simulink model "MLRC_Project_debug"  (R2022a)
settings: Solver=ode45  StartTime=0.0  StopTime=100  RelTol=1e-3  EnableMultiTasking=on
settings Model: Creator=Administrator  LastModifiedBy=rakes
settings DataIOCC: LimitDataPoints=on  SaveFormat=Array  ReturnWorkspaceOutputs=off
settings OptimizationCC: LifeSpan=inf
settings DebuggingCC: SolverPrmCheckMsg=warning  UnconnectedInputMsg=warning  UnconnectedOutputMsg=warning  UnconnectedLineMsg=warning  AllowSymbolicDim=off  SFUnexpectedBacktrackingDiag=warning  SFNoUnconditionalDefaultTransitionDiag=warning  SFExecutionAtInitializationDiag=none  SFMachineParentedDataDiag=warning  ArithmeticOperatorsInVariantConditions=warning
settings HardwareCC: ProdBitPerPointer=32  ProdBitPerSizeT=32  ProdBitPerPtrDiffT=32  ProdLargestAtomicFloat=None  ProdIntDivRoundTo=Undefined  ProdEndianess=Unspecified  ProdWordSize=32  ProdHWDeviceType=32-bit Generic
settings ModelReferenceCC: PropagateSignalLabelsOutOfModel=off
settings SFSimCC: SimUseLocalCustomCode=off  CustomCodeUndefinedFunction=UseInterfaceOnly
settings RTWCC: RTWUseLocalCustomCode=off
settings CodeAppCC: StateflowObjectComments=on
settings GRTTargetCC: TargetLangStandard=C89/C90 (ANSI)
settings ConfigComp: CovMetricSettings=dw  CovSaveCumulativeToWorkspaceVar=on  CovSaveSingleToWorkspaceVar=on  CovExternalEMLEnable=off  CovSFcnEnable=off

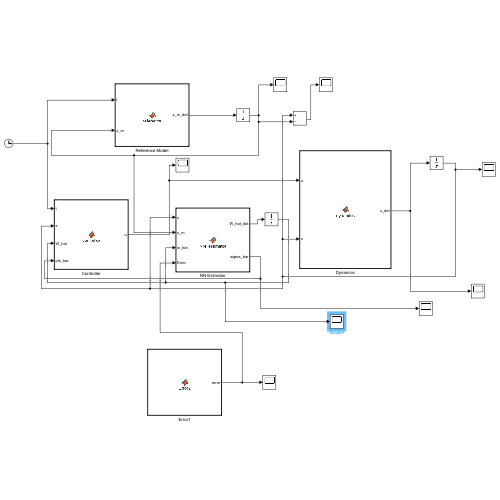
[thumbnail: Simulink's stored preview of the top-level diagram]
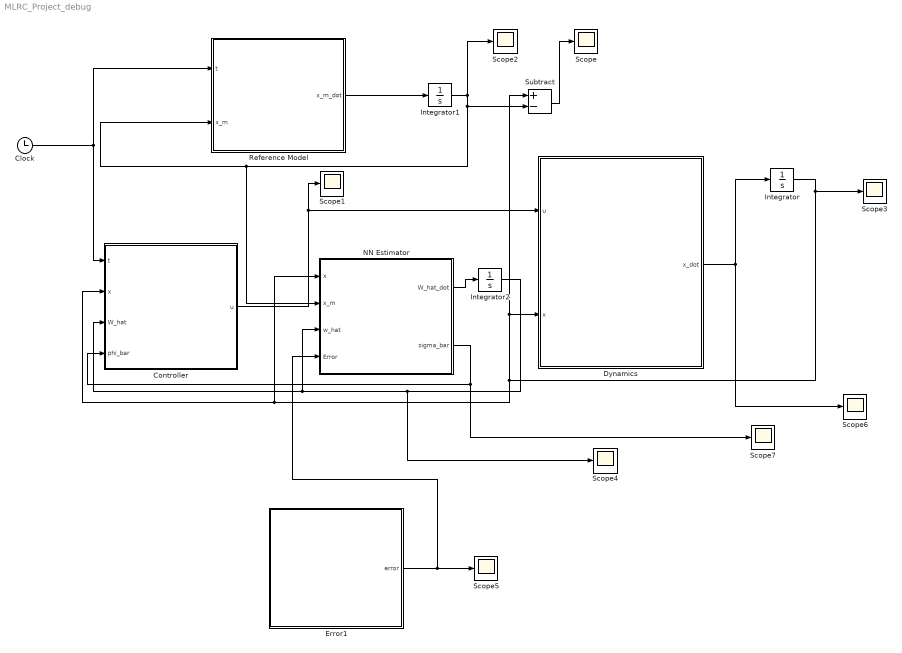
== system MLRC_Project_debug ==
  Clock : Clock
      settings: Decimation=50
  Controller : MATLAB Function  TreatAsAtomicUnit=on
  Dynamics : MATLAB Function  TreatAsAtomicUnit=on
  Error1 : MATLAB Function  TreatAsAtomicUnit=on
  Integrator : Integrator  InitialCondition=[-1;1]
  Integrator1 : Integrator  InitialCondition=[0;0]
  Integrator2 : Integrator  InitialCondition=zeros(6,1)
  NN Estimator : MATLAB Function  TreatAsAtomicUnit=on
  Reference Model : MATLAB Function  TreatAsAtomicUnit=on
  Scope{,1..7} (8 alike) : Scope
  Subtract : Sum  Inputs=+-
  wires:
  Dynamics/1(x_dot) -> Scope6/1, Integrator/1
  Integrator/1 -> Scope3/1, Subtract/1, Dynamics/2(x), NN Estimator/1(x), Controller/2(x)
  Clock/1 -> Controller/1(t), Reference Model/1(t)
  Controller/1(u) -> Scope1/1, Dynamics/1(u)
  Reference Model/1(x_m_dot) -> Integrator1/1
  Integrator1/1 -> Scope2/1, NN Estimator/2(x_m), Reference Model/2(x_m), Subtract/2
  NN Estimator/1(W_hat_dot) -> Integrator2/1
  Integrator2/1 -> Scope4/1, Controller/3(W_hat), NN Estimator/3(w_hat)
  Subtract/1 -> Scope/1
  NN Estimator/2(sigma_bar) -> Scope7/1, Controller/4(phi_bar)
  Error1/1(error) -> NN Estimator/4(Error), Scope5/1

== matlab function MLRC_Project_debug/Controller ==
  data: u output; t input; x input; W_hat input; phi_bar input
function u  = controller(t,x,W_hat, phi_bar)

%r=10;
%r=exp(-t);
r=sin(t);
%r=2*sin(t);

k_x=[-2/3 -1/3]'; % note that the linear control gain is directly chosen instead of adapting with an assumption of $A$ matrix to be known


u=k_x'*x+r-W_hat'*phi_bar;

end

== matlab function MLRC_Project_debug/Dynamics ==
  data: u input; x input; x_dot output
function x_dot   = dynamics(u,x)
%#codegen
L_delta_a=3;
A=[0 1; 0 0];
B=[0;L_delta_a];
W0=0.8;
W1=0.2314;
W2=0.6918;
W3=-0.6245;
W4=0.0095;
W5=0.0214;

theta=x(1,1);
p=x(2,1);

delta=W0+W1*theta+W2*p+W3*abs(theta)*p+W4*abs(p)*p+W5*theta^3;
x_dot=A*x+B*(u+delta/L_delta_a);
end

== matlab function MLRC_Project_debug/NN Estimator ==
  data: W_hat_dot output; x input; x_m input; sigma_bar output; w_hat input; Error input
function [W_hat_dot, sigma_bar]   = NN_estimator(x,x_m, w_hat, Error)

e=x-x_m; % tracking error 

% Omega = [1, 1, 1, 1, 1, 1, 1, 1, 1, 1, 1]';
% Omega = 
L=5; % number of neurons
% L = 10;
Gamma=(3.5)*eye(L+1);
sigma=zeros(L,1);
Vr=5*eye(size(x,1)); % variance of RBF

C=[0.6294   -0.7460    0.2647   -0.4430    0.9150;
    0.8116    0.8268   -0.8049    0.0938    0.9298];  % for L=5

% C=[-0.6848    0.9143    0.6006   -0.1565    0.5844    0.3115    0.6983    0.3575    0.4863    0.3110
%    0.9412   -0.0292   -0.7162    0.8315    0.9190   -0.9286    0.8680    0.5155   -0.2155   -0.6576]; %L=10


for i=1:L
    sigma(i,1)=exp(-((x-C(:,i))'*(Vr\(x-C(:,i)))));
end
sigma_bar=[1;sigma];


P=[3.5 0.5; 0.5 1.5]; % the command P=lyap(A_m',Q) is used to calculate P. In this case Q is chosen as Q=2*eye(2). 
L_delta_a=3;
B=[0;L_delta_a];
% for
% sigma_w = 0.5;
% W_hat_dot=Gamma*sigma_bar*e'*P*B - sigma_w*norm(e)*w_hat;

sigma1_bar = [1 1.783e-01 1.355e-01 7.024e-01 3.249e-01 1.488e-01]';
sigma2_bar = [1 7.663e-01 4.965e-01 2.78e-01 3.766e-01 8.042e-01]';
sigma3_bar = [1 1.448e-01 3.549e-01 4.416e-01 5.083e-01 9.878e-02]';
sigma4_bar = [1 5.883e-01 1.773e-01 4.212e-01 2.701e-01 6.627e-01]';
sigma5_bar = [1 2.908e-01 7.750e-01 2.084e-01 5.632e-01 2.177e-01]';
sigma6_bar = [1 2.195e-01 1.220e-01 7.016e-01 2.963e-01 1.972e-01]';
sigma_star = zeros(6,1,6);
% sigma_star(:, :, 2:6) = 0;
sigma_star(:, :, 1) = [sigma1_bar];
sigma_star(:, :, 2) = [sigma2_bar];
sigma_star(:, :, 3) = [sigma3_bar];
sigma_star(:, :, 4) = [sigma4_bar];
sigma_star(:, :, 5) = [sigma5_bar];
sigma_star(:, :, 6) = [sigma6_bar];

Omega = zeros(L+1, 1, 6);
for i = 1:L+1
    Omega(:, :, i) = sigma_star(:, :, i)*(Error(1, i) - w_hat'*sigma_star(:, :, i));
%     Omega(:, :, i) = sigma_star(:, :, i)*(Error(1, i));

end
% Omega = [sigma1_bar]
Omega_Summation = zeros(6,1);
% for i=1:6
%     Omega_Summation(i,1) = Omega_Summation(i,1) + Omega(:, :, i);
% end

W0=0.8;
W1=0.2314;
W2=0.6918;
W3=-0.6245;
W4=0.0095;
W5=0.0214;

W = [W0 W1 W2 W3 W4 W5]';
k1 = (Error(1, 1) - W'*sigma_star(:, :, 1))
k2 = (Error(1, 2) - W'*sigma_star(:, :, 2))
k3 = (Error(1, 3) - W'*sigma_star(:, :, 3))
k4 = (Error(1, 4) - W'*sigma_star(:, :, 4))
k5 = (Error(1, 5) - W'*sigma_star(:, :, 5))
k6 = (Error(1, 6) - W'*sigma_star(:, :, 6))

Omega_Summation(1,1) = Omega_Summation(1,1) + Omega(1, 1, 1) + Omega(1, 1, 2) + Omega(1, 1, 3)+ Omega(1, 1, 4)+ Omega(1, 1, 5)+ Omega(1, 1, 6);
Omega_Summation(2,1) = Omega_Summation(2,1) + Omega(2, 1, 1) + Omega(2, 1, 2) + Omega(2, 1, 3)+ Omega(2, 1, 4)+ Omega(2, 1, 5)+ Omega(2, 1, 6);
Omega_Summation(3,1) = Omega_Summation(3,1) + Omega(3, 1, 1) + Omega(3, 1, 2) + Omega(3, 1, 3)+ Omega(3, 1, 4)+ Omega(3, 1, 5)+ Omega(3, 1, 6);
Omega_Summation(4,1) = Omega_Summation(4,1) + Omega(4, 1, 1) + Omega(4, 1, 2) + Omega(4, 1, 3)+ Omega(4, 1, 4)+ Omega(4, 1, 5)+ Omega(4, 1, 6);
Omega_Summation(5,1) = Omega_Summation(5,1) + Omega(5, 1, 1) + Omega(5, 1, 2) + Omega(5, 1, 3)+ Omega(5, 1, 4)+ Omega(5, 1, 5)+ Omega(5, 1, 6);
Omega_Summation(6,1) = Omega_Summation(6,1) + Omega(6, 1, 1) + Omega(6, 1, 2) + Omega(6, 1, 3)+ Omega(6, 1, 4)+ Omega(6, 1, 5)+ Omega(6, 1, 6);

sigma_w = 0.5;
W_hat_dot=Gamma*sigma_bar*e'*P*B - sigma_w*norm(e)*w_hat + Gamma*Omega_Summation;

% W_hat_dot=Gamma*sigma_bar*e'*P*B - sigma_w*norm(e)*w_hat;

== matlab function MLRC_Project_debug/Reference Model ==
  data: x_m_dot output; t input; x_m input
function x_m_dot  = reference(t,x_m)
am1=-2;
am2=-1;
L_delta_a=3;
%r=exp(-t);
r=sin(t);
%r=2*sin(t);
A_m=[0 1; am1 am2];
B_m=[0; L_delta_a];
x_m_dot=A_m*x_m+B_m*r;

== matlab function MLRC_Project_debug/Error1 ==
  data: error output
function error = Error2
% function error = Error2(x_dot, x, u, sigma_bar)
% function error = Error2(x_dot, x, u, sigma_bar)

A=[0 1; 0 0];
B=[0;3];

W0=0.8;
W1=0.2314;
W2=0.6918;
W3=-0.6245;
W4=0.0095;
W5=0.0214;

W = [W0 W1 W2 W3 W4 W5];

% error = x_dot/B - A*x/B - u - W*sigma_bar;
u_1 = -1.055e-01;
u_2 = -5.645e-01;
u_3 = 3.984e-01;
u_4 = -1.063e+00;
u_5 = 1.120e-01;
u_6 = -6.223e-01;

x1 = [4.068e-01;
      -2.111e+00];

x2 = [7.465e-01;
      1.954e+00];

x3 = [-1.705e+00;
       -1.235e+00];

x4 = [2.114e+00;
      1.442e-01];

x5 = [-1.481e+00;
       1.033e+00];

x6 = [9.734e-01;
      -1.917e+00];

x1_dot = [-2.111e+00;
           -3.917e-01];
x2_dot = [1.954e+00;
          -2.322e-01];

x3_dot = [-1.2353e+00;
           1.931e+00];

x4_dot = [1.442e-01;
           1.787e+00];

x5_dot = [1.033e+00;
           1.921e+00];

x6_dot = [-1.917e+00;
           -1.025e+00];


sigma1_bar = [1 1.783e-01 1.355e-01 7.024e-01 3.249e-01 1.488e-01]';
sigma2_bar = [1 7.663e-01 4.965e-01 2.78e-01 3.766e-01 8.042e-01]';
sigma3_bar = [1 1.448e-01 3.549e-01 4.416e-01 5.083e-01 9.878e-02]';
sigma4_bar = [1 5.883e-01 1.773e-01 4.212e-01 2.701e-01 6.627e-01]';
sigma5_bar = [1 2.908e-01 7.750e-01 2.084e-01 5.632e-01 2.177e-01]';
sigma6_bar = [1 2.195e-01 1.220e-01 7.016e-01 2.963e-01 1.972e-01]';

error = zeros(1,6);
error(1) = inv(B'*B)*B'*x1_dot - inv(B'*B)*B'*A*x1 - u_1 - W*sigma1_bar;
error(2) = inv(B'*B)*B'*x2_dot - inv(B'*B)*B'*A*x2 - u_2 - W*sigma2_bar;
error(3) = inv(B'*B)*B'*x3_dot - inv(B'*B)*B'*A*x3 - u_3 - W*sigma3_bar;
error(4) = inv(B'*B)*B'*x4_dot - inv(B'*B)*B'*A*x4 - u_4 - W*sigma4_bar;
error(5) = inv(B'*B)*B'*x5_dot - inv(B'*B)*B'*A*x5 - u_5 - W*sigma5_bar;
error(6) = inv(B'*B)*B'*x6_dot - inv(B'*B)*B'*A*x6 - u_6 - W*sigma6_bar;

% syms error(1)
% eqn1 = x1_dot == A*x1 + B*(u_1 + W*sigma1_bar);
% Sol1 = solve(eqn1, error(1));
% 
% syms error(2)
% eqn2 = x2_dot == A*x2 + B*(u_2 + W*sigma2_bar);
% Sol2 = solve(eqn2, error(2))
% 
% syms error(3)
% eqn3 = x3_dot == A*x3 + B*(u_3 + W*sigma3_bar);
% Sol3 = solve(eqn3, error(3))
% 
% syms error(4)
% eqn4 = x4_dot == A*x4 + B*(u_4 + W*sigma4_bar);
% Sol4 = solve(eqn4, error(4))
% 
% syms error(5)
% eqn5 = x5_dot == A*x5 + B*(u_5 + W*sigma5_bar);
% Sol5 = solve(eqn5, error(5))
% 
% syms error(6)
% eqn6 = x6_dot == A*x6 + B*(u_6 + W*sigma6_bar);
% Sol6 = solve(eqn6, error(6))

error = [error(1) error(2) error(3) error(4) error(5) error(6)];
% error =1;
